simulink model "KSimulator_robot"  (Simulink 9.0)
settings: Solver=FixedStepDiscrete  StartTime=0.0  StopTime=5  FixedStep=0.01  RelTol=1e-3  EnableMultiTasking=on
undefined symbols (not defined in the file or in its folder): FK_Robot
settings Model: SuppressorTable=22 serialization::archive 11 0 6 0 0 0 11 0  Creator=E. Dean  LastModifiedBy=nirnai
settings DataIOCC: LimitDataPoints=on  SignalLoggingSaveFormat=ModelDataLogs
settings OptimizationCC: ExpressionDepthLimit=2147483647
settings DebuggingCC: SolverPrmCheckMsg=warning  FcnCallInpInsideContextMsg=warning  StateNameClashWarn=warning
settings GRTTargetCC: GeneratePreprocessorConditionals=Disable all  CombineOutputUpdateFcns=off  GRTInterface=on

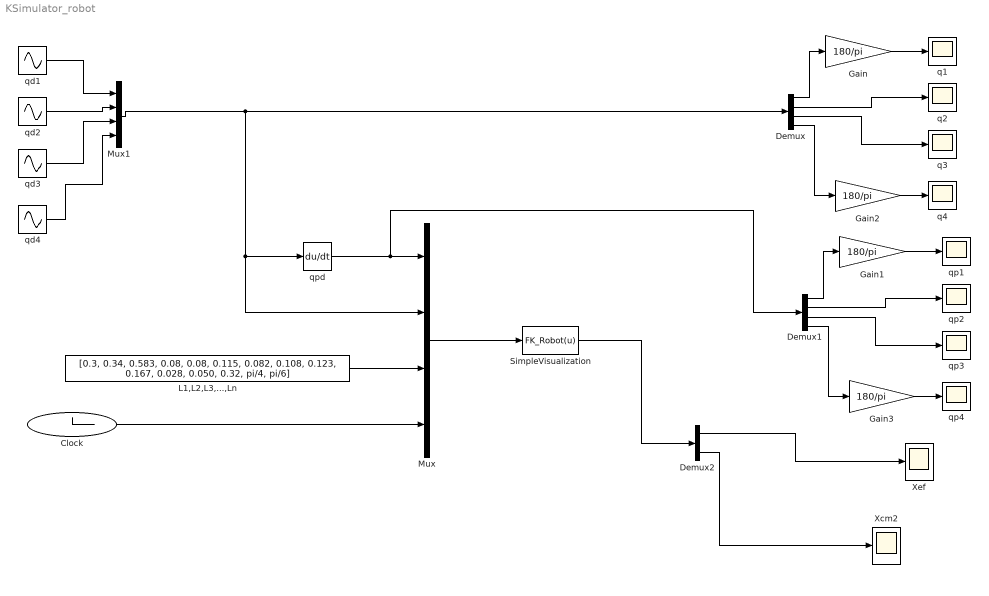
== system KSimulator_robot ==
  Clock : Clock
  Demux : Demux
  Demux1 : Demux
  Demux2 : Demux  Outputs=2
  Gain{,1..3} (4 alike) : Gain  Gain=180/pi
  L1,L2,L3,...,Ln : Constant  Value=[0.3, 0.34, 0.583, 0.08, 0.08, 0.115, 0.082, 0.108, 0.123, 0.167, 0.028, 0.050, 0.32, pi/4, pi/6]
  Mux : Mux
  Mux1 : Mux
  SimpleVisualization : MATLABFcn  MATLABFcn=FK_Robot(u)  OutputDimensions=6
  Xcm2 : Scope
  Xef : Scope
  q{1..4} (4 alike) : Scope
  qd1 : Sin  Amplitude=pi  SampleTime=0
  qd2 : Sin  Amplitude=0.1  Bias=0.1529  SampleTime=0
  qd3 : Sin  Amplitude=0.1  Bias=0.1529  SampleTime=0
  qd4 : Sin  Amplitude=pi  SampleTime=0
  qp{1..4} (4 alike) : Scope
  qpd : Derivative
  wires:
  Demux/2 -> q2/1
  Mux/1 -> SimpleVisualization/1
  Demux/3 -> q3/1
  qd1/1 -> Mux1/1
  qd2/1 -> Mux1/2
  qd3/1 -> Mux1/3
  Mux1/1 -> qpd/1, Mux/2, Demux/1
  qpd/1 -> Demux1/1, Mux/1
  SimpleVisualization/1 -> Demux2/1
  Demux2/1 -> Xef/1
  Demux2/2 -> Xcm2/1
  qd4/1 -> Mux1/4
  Demux/1 -> Gain/1
  Gain/1 -> q1/1
  Gain2/1 -> q4/1
  Demux/4 -> Gain2/1
  Demux1/1 -> Gain1/1
  Gain3/1 -> qp4/1
  Gain1/1 -> qp1/1
  Demux1/2 -> qp2/1
  Demux1/4 -> Gain3/1
  Demux1/3 -> qp3/1
  Clock/1 -> Mux/4
  L1,L2,L3,...,Ln/1 -> Mux/3
